simulink model "malt"  (R2022a)
settings: Solver=FixedStepAuto  StartTime=0.0  StopTime=50  FixedStep=framePeriod_s  RelTol=1e-3
undefined symbols (not defined in the file): Aircraft, DiscIntNeverNeededParam, framePeriod_s, frameRate_hz
libraries: simulink x46, slpidlib x16, dspmathops x1
(part 3 of 4)

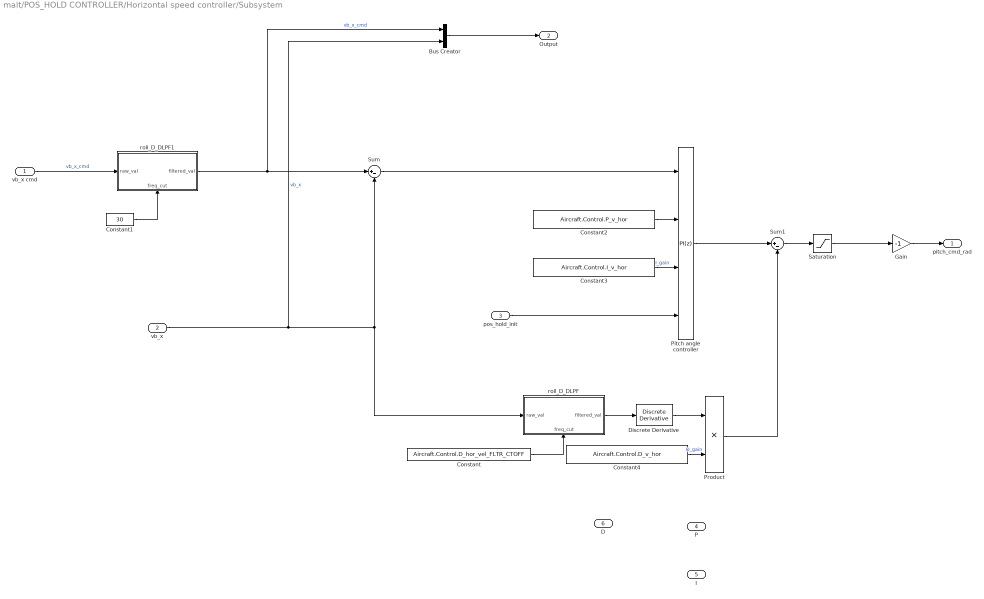
== system malt/POS_HOLD CONTROLLER/Horizontal speed controller/Subsystem ==
  vb_x cmd : Inport
  vb_x : Inport  Port=2
  pos_hold_init : Inport  Port=3
  P : Inport  Port=4
  I : Inport  Port=5
  D : Inport  Port=6
  Bus Creator : BusCreator  Inputs=2
  Constant : Constant  Value=Aircraft.Control.D_hor_vel_FLTR_CTOFF  OutDataTypeStr=single
  Constant1 : Constant  Value=30  OutDataTypeStr=single
  Constant2 : Constant  Value=Aircraft.Control.P_v_hor  OutDataTypeStr=single
  Constant3 : Constant  Value=Aircraft.Control.I_v_hor  OutDataTypeStr=single
  Constant4 : Constant  Value=Aircraft.Control.D_v_hor  OutDataTypeStr=single
  Discrete Derivative : simulink/Discrete/Discrete Derivative  gainval=1.0  ICPrevScaledInput=0.0  OutMin=[]  OutMax=[]  OutDataType=fixdt(1, 16)  OutScaling=2^-10  DoSatur=off
  Gain : Gain  Gain=-1
  Pitch angle controller : slpidlib/PID Controller  Controller=PI  Form=Parallel  TimeDomain=Discrete-time  UseExternalTs=off  SampleTime=framePeriod_s  IntegratorMethod=Forward Euler  FilterMethod=Forward Euler  ControllerParametersSource=external  P=0.335  I=0.005  UseKiTs=off  D=0  N=100  UseFilter=off  TunerSelectOption=Transfer Function Based (PID Tuner App)  InitialConditionSource=internal  InitialConditionForIntegrator=0  InitialConditionForFilter=0  DifferentiatorICPrevScaledInput=0  ExternalReset=either  TrackingMode=off  Kt=1  LimitOutput=on  SatLimitsSource=internal  UpperSaturationLimit=Aircraft.Control.pitch_angle_lim  LowerSaturationLimit=-Aircraft.Control.pitch_angle_lim  LinearizeAsGain=off  AntiWindupMode=clamping  Kb=1  POutMin=[]  POutMax=[]  IOutMin=[]  IOutMax=[]  DOutMin=[]  DOutMax=[]  NOutMin=[]  NOutMax=[]  SumOutMin=[]  SumOutMax=[]  SaturationOutMin=[]  SaturationOutMax=[]  PParamMin=[]  PParamMax=[]  IParamMin=[]  IParamMax=[]  DParamMin=[]  DParamMax=[]  NParamMin=[]  NParamMax=[]  KbParamMin=[]  KbParamMax=[]  KtParamMin=[]  KtParamMax=[]  KbOutMin=[]  KbOutMax=[]  KtOutMin=[]  KtOutMax=[]  IntegratorOutMin=[]  IntegratorOutMax=[]  FilterOutMin=[]  FilterOutMax=[]  SumI1OutMin=[]  SumI1OutMax=[]  SumI2OutMin=[]  SumI2OutMax=[]  SumI3OutMin=[]  SumI3OutMax=[]  SumI4OutMin=[]  SumI4OutMax=[]  SumDOutMin=[]  SumDOutMax=[]  DifferentiatorOutMin=[]  DifferentiatorOutMax=[]  FilterDiffOutCoefMin=[]  FilterDiffOutCoefMax=[]  ReciprocalOutMin=[]  ReciprocalOutMax=[]  SumDenOutMin=[]  SumDenOutMax=[]  SumNumOutMin=[]  SumNumOutMax=[]  DivideOutMin=[]  DivideOutMax=[]  UdiffTsProdOutMin=[]  UdiffTsProdOutMax=[]  NTsProdOutMin=[]  NTsProdOutMax=[]  UintegralTsProdOutMin=[]  UintegralTsProdOutMax=[]  UngainTsProdOutMin=[]  UngainTsProdOutMax=[]  IntegratorContinuousStateAttributes=''  IntegratorStateMustResolveToSignalObject=off  IntegratorRTWStateStorageClass=Auto  FilterContinuousStateAttributes=''  FilterStateMustResolveToSignalObject=off  FilterRTWStateStorageClass=Auto  ParallelPVariant=ExternalParameters  IdealPVariant=Disabled  IVariant=ExternalParameters  DVariant=Disabled  IntegratorVariant=Discrete  SatVariant=Enabled  AWVariant=DiscClampingParallel  PCopyVariant=Disabled  TRVariant=Disabled  FdbkBlocksVariant=Forward  IdealPFdbkVariant=Disabled  SatFdbkVariant=Disabled  DerivativeFilterVariant=Disabled  NVariant=Disabled  NCopyVariant=Disabled_SignalSpec  FilterICVariant=Disabled  IntegratorICVariant=InternalICs  ExternalResetVariant=ExternalReset  TRSumVariant=Passthrough  SumFdbkVariant=Disabled  SumVariant=Sum_PI  TsampFilterVariant=InternalTs  TsampNgainVariant=Passthrough  TsampIntegralVariant=Passthrough  ExternalSaturationOutDataTypeStr=Inherit: Same as second input  aMode=0
  Product : Product
  Saturation : Saturate  UpperLimit=Aircraft.Control.pitch_angle_lim  LowerLimit=-Aircraft.Control.pitch_angle_lim  LinearizeAsGain=off
  Sum : Sum  Inputs=|+-
  Sum1 : Sum  Inputs=|+-
  roll_D_DLPF : Subsystem
      settings: PortSchema="{\"entries\":[{\"content\":{\"sides\":[{\"content\":{\"connectorIds\":[\"In1\"]},\"type\":\"ConnectorPlacement.EquallySpacedRectSide\",\"uuid\":\"20236834-aeb3-4c5b-bb2e-f84447e752b5\"},{\"content\":{\"connectorIds\":[\"Out1\"],\"side\":\"RIGHT\"},\"type\":\"ConnectorPlacement.EquallySpacedRectSide\",\"uuid\":\"d668f9a1-a3df-4207-8bf1-99fb838e59b2\"},{\"content\":{\"connectorIds\":[],\"side\":\"TOP\"},\"type\":\"ConnectorPlacement.EquallySpacedRectSide\",\"uuid\":\"66cceb06-f4bc-4278-b965-2427292e46df\"},{\"content\":{\"connectorIds\":[\"In2\"],\"side\":\"BOTTOM\"},\"type\":\"ConnectorPlacement.EquallySpacedRectSide\",\"uuid\":\"8fdaac6a-cb03-4bd4-87bb-7bafd10bc297\"}]},\"type\":\"ConnectorPlacement.EquallySpacedConnector\",\"uuid\":\"3dc29a9a-e794-478d-b7df-452e6c2d3f66\"}],\"packageUris\":[\"http://schema.mathworks.com/mf0/Connector/R2020b\"],\"version\":\"1.0\"}"
  roll_D_DLPF1 : Subsystem
      settings: PortSchema="{\"entries\":[{\"content\":{\"sides\":[{\"content\":{\"connectorIds\":[\"In1\"]},\"type\":\"ConnectorPlacement.EquallySpacedRectSide\",\"uuid\":\"20236834-aeb3-4c5b-bb2e-f84447e752b5\"},{\"content\":{\"connectorIds\":[\"Out1\"],\"side\":\"RIGHT\"},\"type\":\"ConnectorPlacement.EquallySpacedRectSide\",\"uuid\":\"d668f9a1-a3df-4207-8bf1-99fb838e59b2\"},{\"content\":{\"connectorIds\":[],\"side\":\"TOP\"},\"type\":\"ConnectorPlacement.EquallySpacedRectSide\",\"uuid\":\"66cceb06-f4bc-4278-b965-2427292e46df\"},{\"content\":{\"connectorIds\":[\"In2\"],\"side\":\"BOTTOM\"},\"type\":\"ConnectorPlacement.EquallySpacedRectSide\",\"uuid\":\"8fdaac6a-cb03-4bd4-87bb-7bafd10bc297\"}]},\"type\":\"ConnectorPlacement.EquallySpacedConnector\",\"uuid\":\"3dc29a9a-e794-478d-b7df-452e6c2d3f66\"}],\"packageUris\":[\"http://schema.mathworks.com/mf0/Connector/R2020b\"],\"version\":\"1.0\"}"
  pitch_cmd_rad : Outport
  Output : Outport  Port=2
  wires:
  vb_x/1 -> Bus Creator/2, roll_D_DLPF/1(raw_val), Sum/2  "vb_x"
  Sum/1 -> Pitch angle controller/1
  Saturation/1 -> Gain/1
  Gain/1 -> pitch_cmd_rad/1
  pos_hold_init/1 -> Pitch angle controller/4
  Discrete Derivative/1 -> Product/1
  Constant/1 -> roll_D_DLPF/2(freq_cut)
  roll_D_DLPF/1(filtered_val) -> Discrete Derivative/1
  Pitch angle controller/1 -> Sum1/1
  Sum1/1 -> Saturation/1
  Product/1 -> Sum1/2
  Bus Creator/1 -> Output/1
  vb_x cmd/1 -> roll_D_DLPF1/1(raw_val)  "vb_x_cmd"
  roll_D_DLPF1/1(filtered_val) -> Sum/1, Bus Creator/1  "vb_x_cmd"
  Constant1/1 -> roll_D_DLPF1/2(freq_cut)
  Constant4/1 -> Product/2  "D_gain"
  Constant2/1 -> Pitch angle controller/2
  Constant3/1 -> Pitch angle controller/3  "I_gain"

== system malt/POS_HOLD CONTROLLER/Horizontal speed controller/Subsystem1 ==
  vb_y cmd : Inport
  vb_y : Inport  Port=2
  pos_hold_init : Inport  Port=3
  P : Inport  Port=4
  I : Inport  Port=5
  D : Inport  Port=6
  Bus Creator : BusCreator  Inputs=2
  Constant : Constant  Value=Aircraft.Control.D_hor_vel_FLTR_CTOFF  OutDataTypeStr=single
  Constant1 : Constant  Value=30  OutDataTypeStr=single
  Constant2 : Constant  Value=Aircraft.Control.P_v_hor  OutDataTypeStr=single
  Constant3 : Constant  Value=Aircraft.Control.I_v_hor  OutDataTypeStr=single
  Constant5 : Constant  Value=Aircraft.Control.D_v_hor  OutDataTypeStr=single
  Discrete Derivative : simulink/Discrete/Discrete Derivative  gainval=1.0  ICPrevScaledInput=0.0  OutMin=[]  OutMax=[]  OutDataType=fixdt(1, 16)  OutScaling=2^-10  DoSatur=off
  Product : Product
  Roll angle controller : slpidlib/PID Controller  Controller=PI  Form=Parallel  TimeDomain=Discrete-time  UseExternalTs=off  SampleTime=framePeriod_s  IntegratorMethod=Forward Euler  FilterMethod=Forward Euler  ControllerParametersSource=external  P=0.335  I=0.005  UseKiTs=off  D=0  N=100  UseFilter=off  TunerSelectOption=Transfer Function Based (PID Tuner App)  InitialConditionSource=internal  InitialConditionForIntegrator=0  InitialConditionForFilter=0  DifferentiatorICPrevScaledInput=0  ExternalReset=either  TrackingMode=off  Kt=1  LimitOutput=on  SatLimitsSource=internal  UpperSaturationLimit=Aircraft.Control.roll_angle_lim  LowerSaturationLimit=-Aircraft.Control.roll_angle_lim  LinearizeAsGain=off  AntiWindupMode=clamping  Kb=1  POutMin=[]  POutMax=[]  IOutMin=[]  IOutMax=[]  DOutMin=[]  DOutMax=[]  NOutMin=[]  NOutMax=[]  SumOutMin=[]  SumOutMax=[]  SaturationOutMin=[]  SaturationOutMax=[]  PParamMin=[]  PParamMax=[]  IParamMin=[]  IParamMax=[]  DParamMin=[]  DParamMax=[]  NParamMin=[]  NParamMax=[]  KbParamMin=[]  KbParamMax=[]  KtParamMin=[]  KtParamMax=[]  KbOutMin=[]  KbOutMax=[]  KtOutMin=[]  KtOutMax=[]  IntegratorOutMin=[]  IntegratorOutMax=[]  FilterOutMin=[]  FilterOutMax=[]  SumI1OutMin=[]  SumI1OutMax=[]  SumI2OutMin=[]  SumI2OutMax=[]  SumI3OutMin=[]  SumI3OutMax=[]  SumI4OutMin=[]  SumI4OutMax=[]  SumDOutMin=[]  SumDOutMax=[]  DifferentiatorOutMin=[]  DifferentiatorOutMax=[]  FilterDiffOutCoefMin=[]  FilterDiffOutCoefMax=[]  ReciprocalOutMin=[]  ReciprocalOutMax=[]  SumDenOutMin=[]  SumDenOutMax=[]  SumNumOutMin=[]  SumNumOutMax=[]  DivideOutMin=[]  DivideOutMax=[]  UdiffTsProdOutMin=[]  UdiffTsProdOutMax=[]  NTsProdOutMin=[]  NTsProdOutMax=[]  UintegralTsProdOutMin=[]  UintegralTsProdOutMax=[]  UngainTsProdOutMin=[]  UngainTsProdOutMax=[]  IntegratorContinuousStateAttributes=''  IntegratorStateMustResolveToSignalObject=off  IntegratorRTWStateStorageClass=Auto  FilterContinuousStateAttributes=''  FilterStateMustResolveToSignalObject=off  FilterRTWStateStorageClass=Auto  ParallelPVariant=ExternalParameters  IdealPVariant=Disabled  IVariant=ExternalParameters  DVariant=Disabled  IntegratorVariant=Discrete  SatVariant=Enabled  AWVariant=DiscClampingParallel  PCopyVariant=Disabled  TRVariant=Disabled  FdbkBlocksVariant=Forward  IdealPFdbkVariant=Disabled  SatFdbkVariant=Disabled  DerivativeFilterVariant=Disabled  NVariant=Disabled  NCopyVariant=Disabled_SignalSpec  FilterICVariant=Disabled  IntegratorICVariant=InternalICs  ExternalResetVariant=ExternalReset  TRSumVariant=Passthrough  SumFdbkVariant=Disabled  SumVariant=Sum_PI  TsampFilterVariant=InternalTs  TsampNgainVariant=Passthrough  TsampIntegralVariant=Passthrough  ExternalSaturationOutDataTypeStr=Inherit: Same as second input  aMode=0
  Saturation : Saturate  UpperLimit=Aircraft.Control.pitch_angle_lim  LowerLimit=-Aircraft.Control.pitch_angle_lim  LinearizeAsGain=off
  Sum : Sum  Inputs=|+-
  Sum1 : Sum  Inputs=|+-
  roll_D_DLPF : Subsystem
      settings: PortSchema="{\"entries\":[{\"content\":{\"sides\":[{\"content\":{\"connectorIds\":[\"In1\"]},\"type\":\"ConnectorPlacement.EquallySpacedRectSide\",\"uuid\":\"20236834-aeb3-4c5b-bb2e-f84447e752b5\"},{\"content\":{\"connectorIds\":[\"Out1\"],\"side\":\"RIGHT\"},\"type\":\"ConnectorPlacement.EquallySpacedRectSide\",\"uuid\":\"d668f9a1-a3df-4207-8bf1-99fb838e59b2\"},{\"content\":{\"connectorIds\":[],\"side\":\"TOP\"},\"type\":\"ConnectorPlacement.EquallySpacedRectSide\",\"uuid\":\"66cceb06-f4bc-4278-b965-2427292e46df\"},{\"content\":{\"connectorIds\":[\"In2\"],\"side\":\"BOTTOM\"},\"type\":\"ConnectorPlacement.EquallySpacedRectSide\",\"uuid\":\"8fdaac6a-cb03-4bd4-87bb-7bafd10bc297\"}]},\"type\":\"ConnectorPlacement.EquallySpacedConnector\",\"uuid\":\"3dc29a9a-e794-478d-b7df-452e6c2d3f66\"}],\"packageUris\":[\"http://schema.mathworks.com/mf0/Connector/R2020b\"],\"version\":\"1.0\"}"
  roll_D_DLPF1 : Subsystem
      settings: PortSchema="{\"entries\":[{\"content\":{\"sides\":[{\"content\":{\"connectorIds\":[\"In1\"]},\"type\":\"ConnectorPlacement.EquallySpacedRectSide\",\"uuid\":\"20236834-aeb3-4c5b-bb2e-f84447e752b5\"},{\"content\":{\"connectorIds\":[\"Out1\"],\"side\":\"RIGHT\"},\"type\":\"ConnectorPlacement.EquallySpacedRectSide\",\"uuid\":\"d668f9a1-a3df-4207-8bf1-99fb838e59b2\"},{\"content\":{\"connectorIds\":[],\"side\":\"TOP\"},\"type\":\"ConnectorPlacement.EquallySpacedRectSide\",\"uuid\":\"66cceb06-f4bc-4278-b965-2427292e46df\"},{\"content\":{\"connectorIds\":[\"In2\"],\"side\":\"BOTTOM\"},\"type\":\"ConnectorPlacement.EquallySpacedRectSide\",\"uuid\":\"8fdaac6a-cb03-4bd4-87bb-7bafd10bc297\"}]},\"type\":\"ConnectorPlacement.EquallySpacedConnector\",\"uuid\":\"3dc29a9a-e794-478d-b7df-452e6c2d3f66\"}],\"packageUris\":[\"http://schema.mathworks.com/mf0/Connector/R2020b\"],\"version\":\"1.0\"}"
  roll_cmd_rad : Outport
  Output : Outport  Port=2
  wires:
  vb_y/1 -> Bus Creator/2, roll_D_DLPF/1(raw_val), Sum/2  "vb_y"
  Sum/1 -> Roll angle controller/1
  Saturation/1 -> roll_cmd_rad/1
  pos_hold_init/1 -> Roll angle controller/4
  Discrete Derivative/1 -> Product/1
  Constant/1 -> roll_D_DLPF/2(freq_cut)
  roll_D_DLPF/1(filtered_val) -> Discrete Derivative/1
  Roll angle controller/1 -> Sum1/1
  Sum1/1 -> Saturation/1
  Product/1 -> Sum1/2
  Bus Creator/1 -> Output/1
  vb_y cmd/1 -> roll_D_DLPF1/1(raw_val)  "vb_x_cmd"
  Constant1/1 -> roll_D_DLPF1/2(freq_cut)
  roll_D_DLPF1/1(filtered_val) -> Sum/1, Bus Creator/1  "vb_y_cmd"
  Constant5/1 -> Product/2  "I_gain"
  Constant2/1 -> Roll angle controller/2
  Constant3/1 -> Roll angle controller/3  "I_gain"

== system malt/POS_HOLD CONTROLLER/Horizontal speed controller/zero_vel_handling ==
  vb_x cmd : Inport
  vb_y_cmd : Inport  Port=2
  pos_e_feedback : Inport  Port=3
  cur_heading_rad : Inport  Port=4
  pos_hold_init : Inport  Port=5
  P : Inport  Port=6
  AND : Logic  IconShape=distinctive  AllPortsSameDT=off  OutDataTypeStr=boolean
  Cast To Single : DataTypeConversion  OutDataTypeStr=single  SaturateOnIntegerOverflow=off  RndMeth=Floor
  Compare To Constant : simulink/Logic and Bit Operations/Compare To Constant  relop===  const=0  OutDataTypeStr=boolean
  Compare To Constant1 : simulink/Logic and Bit Operations/Compare To Constant  relop===  const=0  OutDataTypeStr=boolean
  Detect Change : simulink/Logic and Bit Operations/Detect Change  vinit=0  OutDataTypeStr=boolean
  Horizontal position controller : Subsystem
  Mux : Mux  Inputs=2
  Mux1 : Mux  Inputs=2
  NOT : Logic  Operator=NOT  IconShape=distinctive  AllPortsSameDT=off  OutDataTypeStr=boolean
  OR : Logic  Operator=OR  IconShape=distinctive  AllPortsSameDT=off  OutDataTypeStr=boolean
  Switch : Switch  Criteria=u2 > Threshold  SaturateOnIntegerOverflow=off  InputSameDT=off
  Unit Delay : UnitDelay  SampleTime=-1  HasFrameUpgradeWarning=on
  set_tar_pos when vel_cmd == 0 : Subsystem  TreatAsAtomicUnit=on
  v_cmd : Outport
  tar_pos_pos_hold : Outport  Port=2
  wires:
  Mux/1 -> Switch/1
  vb_y_cmd/1 -> Mux/2, Compare To Constant1/1
  Compare To Constant1/1 -> AND/2
  Switch/1 -> v_cmd/1
  vb_x cmd/1 -> Mux/1, Compare To Constant/1
  Compare To Constant/1 -> AND/1
  NOT/1 -> set_tar_pos when vel_cmd == 0/Enable, Switch/2
  pos_e_feedback/1 -> set_tar_pos when vel_cmd == 0/1(pos_xy_m), Horizontal position controller/2(cur_pos_m)
  Horizontal position controller/1(vb_x_cmd_mps) -> Mux1/1  "vb_x_cmd_mps"
  Horizontal position controller/2(vb_y_cmd_mps) -> Mux1/2  "vb_y_cmd_mps"
  cur_heading_rad/1 -> Horizontal position controller/3(cur_heading_rad)
  Mux1/1 -> Cast To Single/1
  Cast To Single/1 -> Switch/3
  OR/1 -> NOT/1
  AND/1 -> OR/1
  pos_hold_init/1 -> Unit Delay/1
  Detect Change/1 -> OR/2
  Unit Delay/1 -> Detect Change/1
  set_tar_pos when vel_cmd == 0/1(target_pos_xy_m) -> tar_pos_pos_hold/1, Horizontal position controller/1(cur_target_pos_m)
  P/1 -> Horizontal position controller/4(P)

== system malt/POS_HOLD CONTROLLER/Vertical speed controller/Pitch_D_DLPF ==
  raw_val : Inport
  freq_cut : Inport  Port=2
  MATLAB Function : MATLAB Function  TreatAsAtomicUnit=on
  Unit Delay : UnitDelay  SampleTime=-1  HasFrameUpgradeWarning=on
  filtered_val : Outport
  wires:
  MATLAB Function/1(filtered_val) -> filtered_val/1, Unit Delay/1
  raw_val/1 -> MATLAB Function/2(raw_val)
  Unit Delay/1 -> MATLAB Function/1(prev_val)
  freq_cut/1 -> MATLAB Function/3(freq_cut)

== system malt/POS_HOLD CONTROLLER/Vertical speed controller/Vertical position controller ==
  cur_alt : Inport
  tar_z : Inport  Port=2
  P_alt : Inport  Port=3
  Altitude PID : slpidlib/PID Controller  Controller=P  Form=Ideal  TimeDomain=Discrete-time  UseExternalTs=off  SampleTime=framePeriod_s  IntegratorMethod=Forward Euler  FilterMethod=Forward Euler  ControllerParametersSource=external  P=0  I=0  UseKiTs=off  D=0  N=100  UseFilter=off  TunerSelectOption=Frequency Response Based  ZeroCross=off  InitialConditionSource=internal  InitialConditionForIntegrator=0  InitialConditionForFilter=0  DifferentiatorICPrevScaledInput=0  ExternalReset=either  TrackingMode=off  Kt=1  LimitOutput=on  SatLimitsSource=internal  UpperSaturationLimit=Aircraft.Control.v_z_up_max  LowerSaturationLimit=-Aircraft.Control.v_z_down_max  LinearizeAsGain=on  AntiWindupMode=clamping  Kb=1  POutMin=[]  POutMax=[]  IOutMin=[]  IOutMax=[]  DOutMin=[]  DOutMax=[]  NOutMin=[]  NOutMax=[]  SumOutMin=[]  SumOutMax=[]  SaturationOutMin=[]  SaturationOutMax=[]  PParamMin=[]  PParamMax=[]  IParamMin=[]  IParamMax=[]  DParamMin=[]  DParamMax=[]  NParamMin=[]  NParamMax=[]  KbParamMin=[]  KbParamMax=[]  KtParamMin=[]  KtParamMax=[]  KbOutMin=[]  KbOutMax=[]  KtOutMin=[]  KtOutMax=[]  IntegratorOutMin=[]  IntegratorOutMax=[]  FilterOutMin=[]  FilterOutMax=[]  SumI1OutMin=[]  SumI1OutMax=[]  SumI2OutMin=[]  SumI2OutMax=[]  SumI3OutMin=[]  SumI3OutMax=[]  SumI4OutMin=[]  SumI4OutMax=[]  SumDOutMin=[]  SumDOutMax=[]  DifferentiatorOutMin=[]  DifferentiatorOutMax=[]  FilterDiffOutCoefMin=[]  FilterDiffOutCoefMax=[]  ReciprocalOutMin=[]  ReciprocalOutMax=[]  SumDenOutMin=[]  SumDenOutMax=[]  SumNumOutMin=[]  SumNumOutMax=[]  DivideOutMin=[]  DivideOutMax=[]  UdiffTsProdOutMin=[]  UdiffTsProdOutMax=[]  NTsProdOutMin=[]  NTsProdOutMax=[]  UintegralTsProdOutMin=[]  UintegralTsProdOutMax=[]  UngainTsProdOutMin=[]  UngainTsProdOutMax=[]  IntegratorContinuousStateAttributes=''  IntegratorStateMustResolveToSignalObject=off  IntegratorRTWStateStorageClass=Auto  FilterContinuousStateAttributes=''  FilterStateMustResolveToSignalObject=off  FilterRTWStateStorageClass=Auto  ParallelPVariant=ExternalParameters  IdealPVariant=Disabled  IVariant=Disabled  DVariant=Disabled  IntegratorVariant=Disabled  SatVariant=Enabled  AWVariant=Disabled  PCopyVariant=Disabled  TRVariant=Disabled  FdbkBlocksVariant=Forward  IdealPFdbkVariant=Disabled  SatFdbkVariant=Disabled  DerivativeFilterVariant=Disabled  NVariant=Disabled  NCopyVariant=Disabled_SignalSpec  FilterICVariant=Disabled  IntegratorICVariant=Disabled  ExternalResetVariant=Disabled  TRSumVariant=Passthrough  SumFdbkVariant=Disabled  SumVariant=Passthrough_P  TsampFilterVariant=InternalTs  TsampNgainVariant=Passthrough  TsampIntegralVariant=Disabled_SignalSpec  ExternalSaturationOutDataTypeStr=Inherit: Same as second input  aMode=0
  Sum3 : Sum  Inputs=|+-
  ve_z_cmd_mps : Outport
  wires:
  Altitude PID/1 -> ve_z_cmd_mps/1
  tar_z/1 -> Sum3/1  "target_z"
  cur_alt/1 -> Sum3/2
  Sum3/1 -> Altitude PID/1
  P_alt/1 -> Altitude PID/2

== system malt/POS_HOLD CONTROLLER/Vertical speed controller/set_tar_z when ve_z_cmd == 0 ==
  In1 : Inport
  Enable : EnablePort
  tar_z : Outport
  wires:
  In1/1 -> tar_z/1

== system malt/WAYPOINT CONTROLLER1/WP_NAV/Horizontal position controller ==
  Sys_input : Inport
  cur_target_pos_m : Inport  Port=2
  prev_pos_m : Inport  Port=3
  Bus Creator : BusCreator  Inputs=2
  Bus Selector2 : BusSelector  OutputSignals=Aux Ins Data.ned_pos_m,Ins Data.heading_rad
  Horizontal_position_controller : Subsystem
  deviation_calc : MATLAB Function  TreatAsAtomicUnit=on
  "horizontal_error_calculation " : Subsystem
  vb_x_cmd_mps : Outport
  vb_y_cmd_mps : Outport  Port=2
  Output : Outport  Port=3
  Output1 : Outport  Port=4
  wires:
  Horizontal_position_controller/1(vb_x) -> vb_x_cmd_mps/1
  Horizontal_position_controller/2(vb_y) -> vb_y_cmd_mps/1
  Sys_input/1 -> Bus Selector2/1
  "horizontal_error_calculation "/1(dist_to_target_m) -> Horizontal_position_controller/1(dist_to_tar_m)
  "horizontal_error_calculation "/2(bearing_to_tar_rad) -> Horizontal_position_controller/2(bearing_to_tar_rad)
  Bus Selector2/1 -> "horizontal_error_calculation "/2(cur_pos_m), deviation_calc/2(cur_pos)  "<ned_pos_m>"
  Bus Selector2/2 -> Horizontal_position_controller/5(cur_heading_rad)  "<heading_rad>"
  deviation_calc/1(dev_dist_m) -> Horizontal_position_controller/3(dev_dist_m), Bus Creator/1  "dev_dist"
  cur_target_pos_m/1 -> deviation_calc/1(tar_pos), "horizontal_error_calculation "/1(target_pos_m)
  prev_pos_m/1 -> deviation_calc/3(prev_pos)
  deviation_calc/2(dev_bearing_rad) -> Horizontal_position_controller/4(dev_bearing_rad), Bus Creator/2  "dev_bearing"
  Bus Creator/1 -> Output/1
  Horizontal_position_controller/3(dev_output) -> Output1/1

== system malt/WAYPOINT CONTROLLER1/WP_NAV/Vertical position controller ==
  Sys_input : Inport
  max_v_z_mps : Inport  Port=2
  cur_target_pos_m : Inport  Port=3
  Bus Selector6 : BusSelector  OutputSignals=Navigation Filter Data.bfs_ekf.ned_pos_m
  Selector1 : Selector  InputPortWidth=3  IndexOptions=Index vector (dialog)  Indices=3  OutputSizes=1
  select_cur_z : Selector  InputPortWidth=3  IndexOptions=Index vector (dialog)  Indices=3  OutputSizes=1
  vertical_position_controller : Subsystem
  ve_z_cmd_mps : Outport
  wires:
  Sys_input/1 -> Bus Selector6/1
  Bus Selector6/1 -> select_cur_z/1  "<ned_pos_m>"
  vertical_position_controller/1(ve_z_cmd) -> ve_z_cmd_mps/1
  Selector1/1 -> vertical_position_controller/1(target_z_m)  "target_z"
  select_cur_z/1 -> vertical_position_controller/2(cur_z_m)
  cur_target_pos_m/1 -> Selector1/1
  max_v_z_mps/1 -> vertical_position_controller/3(max_v_z_mps)

== system malt/WAYPOINT CONTROLLER1/WP_NAV/heading_controller ==
  Sys_input : Inport
  cur_target_heading_rad : Inport  Port=2
  Bus Selector4 : BusSelector  OutputSignals=Navigation Filter Data.bfs_ekf.heading_rad
  heading_controller : Subsystem
  yaw_rate_cmd_radps : Outport
  wires:
  Sys_input/1 -> Bus Selector4/1
  cur_target_heading_rad/1 -> heading_controller/1(heading_cmd_rad)
  Bus Selector4/1 -> heading_controller/2(<heading_rad>)  "<heading_rad>"
  heading_controller/1(yaw_rate_cmd) -> yaw_rate_cmd_radps/1

== system malt/determine arm and mode selection/Failsafe_management/Radio failsafe ==
  note: Transition to RTL mode
  note: If radio_failsafe is triggered and current_mode is not auto, rtl, land nor motor_state disarmed then RTL mode is triggered
  failsafe : Inport
  manual_mode : Inport  Port=2
  motor_state : Inport  Port=3
  AND1 : Logic  Commented=on  IconShape=distinctive  AllPortsSameDT=off  OutDataTypeStr=boolean
  Compare To Constant : simulink/Logic and Bit Operations/Compare To Constant  Commented=on  relop=~=  const=3  OutDataTypeStr=boolean
  Compare To Constant1 : simulink/Logic and Bit Operations/Compare To Constant  Commented=on  relop=~=  const=4  OutDataTypeStr=boolean
  Compare To Constant2 : simulink/Logic and Bit Operations/Compare To Constant  Commented=on  relop=~=  const=5  OutDataTypeStr=boolean
  NOR : Logic  Commented=on  Operator=NOR  Inputs=4  IconShape=distinctive  AllPortsSameDT=off  OutDataTypeStr=boolean
  NOT : Logic  Commented=on  Operator=NOT  IconShape=distinctive  AllPortsSameDT=off  OutDataTypeStr=boolean
  NOT1 : Logic  Operator=NOT  IconShape=distinctive  AllPortsSameDT=off  OutDataTypeStr=boolean
  Subsystem : Subsystem
  radio_failsafe_enabled : Outport
  wires:
  manual_mode/1 -> Compare To Constant2/1, Compare To Constant1/1, Compare To Constant/1
  Compare To Constant/1 -> NOR/1
  Compare To Constant1/1 -> NOR/2
  Compare To Constant2/1 -> NOR/3
  motor_state/1 -> NOT/1
  NOT/1 -> NOR/4
  failsafe/1 -> Subsystem/1(<inceptor_health>)
  NOR/1 -> AND1/1
  Subsystem/1(inceptor_health_filtered) -> NOT1/1
  NOT1/1 -> radio_failsafe_enabled/1

== system malt/determine arm and mode selection/Subsystem/e_stop counter ==
  note: This is to ensure e_stop event is not triggered unless e_stop command is sent for more than 0.3 s to prevent false trigger
  motor_e_stop_raw : Inport
  Enable : EnablePort  StatesWhenEnabling=reset
  Compare To Constant : simulink/Logic and Bit Operations/Compare To Constant  relop=>=  const=0.5  OutDataTypeStr=boolean
  Discrete-Time Integrator : DiscreteIntegrator  SampleTime=framePeriod_s  LimitOutput=on  UpperSaturationLimit=1  LowerSaturationLimit=0  ICPrevOutput=DiscIntNeverNeededParam  ICPrevScaledInput=DiscIntNeverNeededParam
  Gain : Gain  Gain=2
  e_stop_filtered : Outport
  wires:
  Compare To Constant/1 -> e_stop_filtered/1
  Discrete-Time Integrator/1 -> Compare To Constant/1
  Gain/1 -> Discrete-Time Integrator/1
  motor_e_stop_raw/1 -> Gain/1

== system malt/determine arm and mode selection/yaw_stick_arming/Enabled Subsystem ==
  yaw_input : Inport
  Enable : EnablePort  StatesWhenEnabling=reset
  Cast : DataTypeConversion  OutDataTypeStr=int8  SaturateOnIntegerOverflow=off  RndMeth=Floor
  Discrete-Time Integrator : DiscreteIntegrator  IntegratorMethod=Integration: Trapezoidal  SampleTime=framePeriod_s  OutDataTypeStr=single  UpperSaturationLimit=1  LowerSaturationLimit=0  ICPrevOutput=DiscIntNeverNeededParam  ICPrevScaledInput=DiscIntNeverNeededParam
  time_arm_valid_s : Outport
  wires:
  Discrete-Time Integrator/1 -> time_arm_valid_s/1
  Cast/1 -> Discrete-Time Integrator/1
  yaw_input/1 -> Cast/1

== system malt/determine arm and mode selection/yaw_stick_arming/manual_arming ==
  yaw_arm : Inport
  Trigger : TriggerPort  VariantControl=(inherit)  PortDimensions=1
  arm_state : Outport
  wires:
  yaw_arm/1 -> arm_state/1

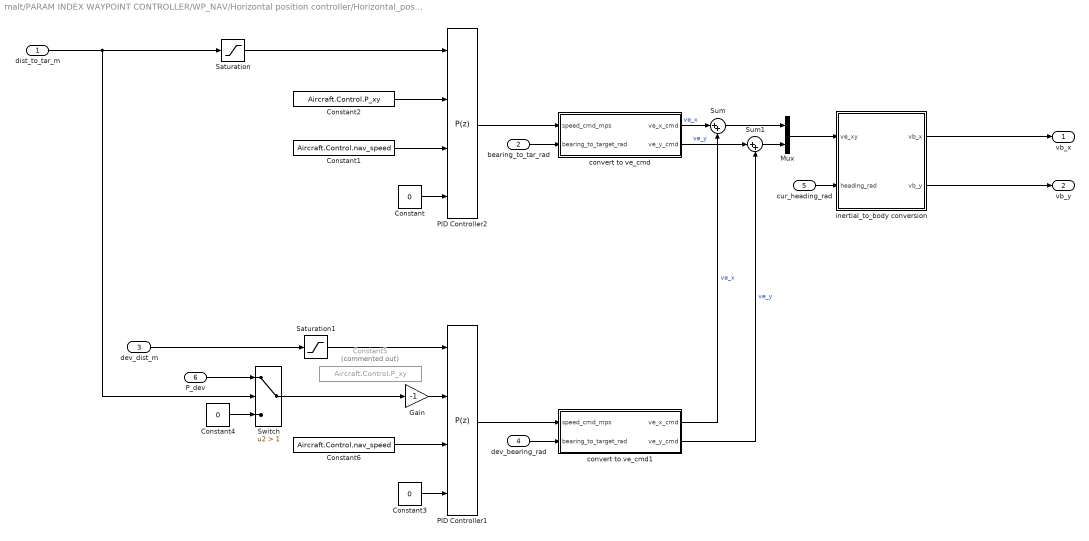
== system malt/PARAM INDEX WAYPOINT CONTROLLER/WP_NAV/Horizontal position controller/Horizontal_position_controller ==
  dist_to_tar_m : Inport
  bearing_to_tar_rad : Inport  Port=2
  dev_dist_m : Inport  Port=3
  dev_bearing_rad : Inport  Port=4
  cur_heading_rad : Inport  Port=5
  P_dev : Inport  Port=6
  Constant : Constant  Value=0  OutDataTypeStr=single
  Constant1 : Constant  Value=Aircraft.Control.nav_speed  OutDataTypeStr=single
  Constant2 : Constant  Value=Aircraft.Control.P_xy  OutDataTypeStr=single
  Constant3 : Constant  Value=0  OutDataTypeStr=single
  Constant4 : Constant  Value=0  OutDataTypeStr=single
  Constant5 : Constant  Commented=on  Value=Aircraft.Control.P_xy  OutDataTypeStr=single
  Constant6 : Constant  Value=Aircraft.Control.nav_speed  OutDataTypeStr=single
  Gain : Gain  Gain=-1
  Mux : Mux  Inputs=2
  PID Controller1 : slpidlib/PID Controller  Controller=P  Form=Parallel  TimeDomain=Discrete-time  UseExternalTs=off  SampleTime=framePeriod_s  IntegratorMethod=Forward Euler  FilterMethod=Forward Euler  ControllerParametersSource=external  P=0.335  I=0.005  UseKiTs=off  D=0  N=100  UseFilter=off  TunerSelectOption=Transfer Function Based (PID Tuner App)  InitialConditionSource=internal  InitialConditionForIntegrator=0  InitialConditionForFilter=0  DifferentiatorICPrevScaledInput=0  ExternalReset=none  TrackingMode=off  Kt=1  LimitOutput=on  SatLimitsSource=external  UpperSaturationLimit=inf  LowerSaturationLimit=-inf  LinearizeAsGain=off  AntiWindupMode=clamping  Kb=1  POutMin=[]  POutMax=[]  IOutMin=[]  IOutMax=[]  DOutMin=[]  DOutMax=[]  NOutMin=[]  NOutMax=[]  SumOutMin=[]  SumOutMax=[]  SaturationOutMin=[]  SaturationOutMax=[]  PParamMin=[]  PParamMax=[]  IParamMin=[]  IParamMax=[]  DParamMin=[]  DParamMax=[]  NParamMin=[]  NParamMax=[]  KbParamMin=[]  KbParamMax=[]  KtParamMin=[]  KtParamMax=[]  KbOutMin=[]  KbOutMax=[]  KtOutMin=[]  KtOutMax=[]  IntegratorOutMin=[]  IntegratorOutMax=[]  FilterOutMin=[]  FilterOutMax=[]  SumI1OutMin=[]  SumI1OutMax=[]  SumI2OutMin=[]  SumI2OutMax=[]  SumI3OutMin=[]  SumI3OutMax=[]  SumI4OutMin=[]  SumI4OutMax=[]  SumDOutMin=[]  SumDOutMax=[]  DifferentiatorOutMin=[]  DifferentiatorOutMax=[]  FilterDiffOutCoefMin=[]  FilterDiffOutCoefMax=[]  ReciprocalOutMin=[]  ReciprocalOutMax=[]  SumDenOutMin=[]  SumDenOutMax=[]  SumNumOutMin=[]  SumNumOutMax=[]  DivideOutMin=[]  DivideOutMax=[]  UdiffTsProdOutMin=[]  UdiffTsProdOutMax=[]  NTsProdOutMin=[]  NTsProdOutMax=[]  UintegralTsProdOutMin=[]  UintegralTsProdOutMax=[]  UngainTsProdOutMin=[]  UngainTsProdOutMax=[]  IntegratorContinuousStateAttributes=''  IntegratorStateMustResolveToSignalObject=off  IntegratorRTWStateStorageClass=Auto  FilterContinuousStateAttributes=''  FilterStateMustResolveToSignalObject=off  FilterRTWStateStorageClass=Auto  ParallelPVariant=ExternalParameters  IdealPVariant=Disabled  IVariant=Disabled  DVariant=Disabled  IntegratorVariant=Disabled  SatVariant=External  AWVariant=Disabled  PCopyVariant=Disabled  TRVariant=Disabled  FdbkBlocksVariant=Forward  IdealPFdbkVariant=Disabled  SatFdbkVariant=Disabled  DerivativeFilterVariant=Disabled  NVariant=Disabled  NCopyVariant=Disabled_SignalSpec  FilterICVariant=Disabled  IntegratorICVariant=Disabled  ExternalResetVariant=Disabled  TRSumVariant=Passthrough  SumFdbkVariant=Disabled  SumVariant=Passthrough_P  TsampFilterVariant=InternalTs  TsampNgainVariant=Passthrough  TsampIntegralVariant=Disabled_SignalSpec  ExternalSaturationOutDataTypeStr=Inherit: Same as second input  aMode=0
  PID Controller2 : slpidlib/PID Controller  Controller=P  Form=Parallel  TimeDomain=Discrete-time  UseExternalTs=off  SampleTime=framePeriod_s  IntegratorMethod=Forward Euler  FilterMethod=Forward Euler  ControllerParametersSource=external  P=0.335  I=0.005  UseKiTs=off  D=0  N=100  UseFilter=off  TunerSelectOption=Transfer Function Based (PID Tuner App)  InitialConditionSource=internal  InitialConditionForIntegrator=0  InitialConditionForFilter=0  DifferentiatorICPrevScaledInput=0  ExternalReset=none  TrackingMode=off  Kt=1  LimitOutput=on  SatLimitsSource=external  UpperSaturationLimit=inf  LowerSaturationLimit=-inf  LinearizeAsGain=off  AntiWindupMode=clamping  Kb=1  POutMin=[]  POutMax=[]  IOutMin=[]  IOutMax=[]  DOutMin=[]  DOutMax=[]  NOutMin=[]  NOutMax=[]  SumOutMin=[]  SumOutMax=[]  SaturationOutMin=[]  SaturationOutMax=[]  PParamMin=[]  PParamMax=[]  IParamMin=[]  IParamMax=[]  DParamMin=[]  DParamMax=[]  NParamMin=[]  NParamMax=[]  KbParamMin=[]  KbParamMax=[]  KtParamMin=[]  KtParamMax=[]  KbOutMin=[]  KbOutMax=[]  KtOutMin=[]  KtOutMax=[]  IntegratorOutMin=[]  IntegratorOutMax=[]  FilterOutMin=[]  FilterOutMax=[]  SumI1OutMin=[]  SumI1OutMax=[]  SumI2OutMin=[]  SumI2OutMax=[]  SumI3OutMin=[]  SumI3OutMax=[]  SumI4OutMin=[]  SumI4OutMax=[]  SumDOutMin=[]  SumDOutMax=[]  DifferentiatorOutMin=[]  DifferentiatorOutMax=[]  FilterDiffOutCoefMin=[]  FilterDiffOutCoefMax=[]  ReciprocalOutMin=[]  ReciprocalOutMax=[]  SumDenOutMin=[]  SumDenOutMax=[]  SumNumOutMin=[]  SumNumOutMax=[]  DivideOutMin=[]  DivideOutMax=[]  UdiffTsProdOutMin=[]  UdiffTsProdOutMax=[]  NTsProdOutMin=[]  NTsProdOutMax=[]  UintegralTsProdOutMin=[]  UintegralTsProdOutMax=[]  UngainTsProdOutMin=[]  UngainTsProdOutMax=[]  IntegratorContinuousStateAttributes=''  IntegratorStateMustResolveToSignalObject=off  IntegratorRTWStateStorageClass=Auto  FilterContinuousStateAttributes=''  FilterStateMustResolveToSignalObject=off  FilterRTWStateStorageClass=Auto  ParallelPVariant=ExternalParameters  IdealPVariant=Disabled  IVariant=Disabled  DVariant=Disabled  IntegratorVariant=Disabled  SatVariant=External  AWVariant=Disabled  PCopyVariant=Disabled  TRVariant=Disabled  FdbkBlocksVariant=Forward  IdealPFdbkVariant=Disabled  SatFdbkVariant=Disabled  DerivativeFilterVariant=Disabled  NVariant=Disabled  NCopyVariant=Disabled_SignalSpec  FilterICVariant=Disabled  IntegratorICVariant=Disabled  ExternalResetVariant=Disabled  TRSumVariant=Passthrough  SumFdbkVariant=Disabled  SumVariant=Passthrough_P  TsampFilterVariant=InternalTs  TsampNgainVariant=Passthrough  TsampIntegralVariant=Disabled_SignalSpec  ExternalSaturationOutDataTypeStr=Inherit: Same as second input  aMode=0
  Saturation : Saturate  UpperLimit=1  LowerLimit=0
  Saturation1 : Saturate  UpperLimit=1  LowerLimit=0
  Sum : Sum  Inputs=|++
  Sum1 : Sum  Inputs=|++
  Switch : Switch  Criteria=u2 > Threshold  Threshold=1  SaturateOnIntegerOverflow=off  InputSameDT=off
  convert to ve_cmd : Subsystem
  convert to ve_cmd1 : Subsystem
  inertial_to_body conversion : Subsystem
  vb_x : Outport
  vb_y : Outport  Port=2
  wires:
  Constant2/1 -> PID Controller2/2
  bearing_to_tar_rad/1 -> convert to ve_cmd/2(bearing_to_target_rad)
  Mux/1 -> inertial_to_body conversion/1(ve_xy)
  Constant1/1 -> PID Controller2/3
  Constant/1 -> PID Controller2/4
  Saturation/1 -> PID Controller2/1
  dist_to_tar_m/1 -> Saturation/1, Switch/2
  cur_heading_rad/1 -> inertial_to_body conversion/2(heading_rad)
  PID Controller2/1 -> convert to ve_cmd/1(speed_cmd_mps)
  inertial_to_body conversion/1(vb_x) -> vb_x/1
  inertial_to_body conversion/2(vb_y) -> vb_y/1
  dev_dist_m/1 -> Saturation1/1
  PID Controller1/1 -> convert to ve_cmd1/1(speed_cmd_mps)
  dev_bearing_rad/1 -> convert to ve_cmd1/2(bearing_to_target_rad)
  Saturation1/1 -> PID Controller1/1
  Constant3/1 -> PID Controller1/4
  Constant6/1 -> PID Controller1/3
  convert to ve_cmd/1(ve_x_cmd) -> Sum/1  "ve_x"
  Sum/1 -> Mux/1
  convert to ve_cmd/2(ve_y_cmd) -> Sum1/1  "ve_y"
  Sum1/1 -> Mux/2
  convert to ve_cmd1/1(ve_x_cmd) -> Sum/2  "ve_x"
  convert to ve_cmd1/2(ve_y_cmd) -> Sum1/2  "ve_y"
  Gain/1 -> PID Controller1/2
  Switch/1 -> Gain/1
  P_dev/1 -> Switch/1
  Constant4/1 -> Switch/3

== system malt/PARAM INDEX WAYPOINT CONTROLLER/WP_NAV/Horizontal position controller/horizontal_error_calculation  ==
  target_pos_m : Inport
  cur_pos_m : Inport  Port=2
  Atan2 : Trigonometry  Operator=atan2
  Demux2 : Demux  Outputs=2
  MatrixMultiply : Product  Multiplication=Matrix(*)
  Selector : Selector  InputPortWidth=3  IndexOptions=Index vector (dialog)  Indices=[1 2]  OutputSizes=1
  Sqrt : Sqrt
  Subtract : Sum  Inputs=+-
  Transpose : Math  Operator=transpose
  dist_to_target_m : Outport
  bearing_to_tar_rad : Outport  Port=2
  wires:
  target_pos_m/1 -> Subtract/1
  cur_pos_m/1 -> Subtract/2
  Selector/1 -> Demux2/1, MatrixMultiply/2, Transpose/1
  Atan2/1 -> bearing_to_tar_rad/1
  Subtract/1 -> Selector/1
  Demux2/2 -> Atan2/1
  Transpose/1 -> MatrixMultiply/1
  MatrixMultiply/1 -> Sqrt/1
  Demux2/1 -> Atan2/2
  Sqrt/1 -> dist_to_target_m/1

== system malt/PARAM INDEX WAYPOINT CONTROLLER/WP_NAV/Vertical position controller/vertical_position_controller ==
  target_z_m : Inport
  cur_z_m : Inport  Port=2
  max_v_z_mps : Inport  Port=3
  Altitude PID : slpidlib/PID Controller  Controller=PI  Form=Ideal  TimeDomain=Discrete-time  UseExternalTs=off  SampleTime=framePeriod_s  IntegratorMethod=Forward Euler  FilterMethod=Forward Euler  ControllerParametersSource=external  P=0  I=0  UseKiTs=off  D=0  N=100  UseFilter=off  TunerSelectOption=Frequency Response Based  ZeroCross=off  InitialConditionSource=internal  InitialConditionForIntegrator=0  InitialConditionForFilter=0  DifferentiatorICPrevScaledInput=0  ExternalReset=none  TrackingMode=off  Kt=1  LimitOutput=on  SatLimitsSource=external  UpperSaturationLimit=Aircraft.Control.v_z_up_max  LowerSaturationLimit=-Aircraft.Control.v_z_down_max  LinearizeAsGain=on  AntiWindupMode=clamping  Kb=1  POutMin=[]  POutMax=[]  IOutMin=[]  IOutMax=[]  DOutMin=[]  DOutMax=[]  NOutMin=[]  NOutMax=[]  SumOutMin=[]  SumOutMax=[]  SaturationOutMin=[]  SaturationOutMax=[]  PParamMin=[]  PParamMax=[]  IParamMin=[]  IParamMax=[]  DParamMin=[]  DParamMax=[]  NParamMin=[]  NParamMax=[]  KbParamMin=[]  KbParamMax=[]  KtParamMin=[]  KtParamMax=[]  KbOutMin=[]  KbOutMax=[]  KtOutMin=[]  KtOutMax=[]  IntegratorOutMin=[]  IntegratorOutMax=[]  FilterOutMin=[]  FilterOutMax=[]  SumI1OutMin=[]  SumI1OutMax=[]  SumI2OutMin=[]  SumI2OutMax=[]  SumI3OutMin=[]  SumI3OutMax=[]  SumI4OutMin=[]  SumI4OutMax=[]  SumDOutMin=[]  SumDOutMax=[]  DifferentiatorOutMin=[]  DifferentiatorOutMax=[]  FilterDiffOutCoefMin=[]  FilterDiffOutCoefMax=[]  ReciprocalOutMin=[]  ReciprocalOutMax=[]  SumDenOutMin=[]  SumDenOutMax=[]  SumNumOutMin=[]  SumNumOutMax=[]  DivideOutMin=[]  DivideOutMax=[]  UdiffTsProdOutMin=[]  UdiffTsProdOutMax=[]  NTsProdOutMin=[]  NTsProdOutMax=[]  UintegralTsProdOutMin=[]  UintegralTsProdOutMax=[]  UngainTsProdOutMin=[]  UngainTsProdOutMax=[]  IntegratorContinuousStateAttributes=''  IntegratorStateMustResolveToSignalObject=off  IntegratorRTWStateStorageClass=Auto  FilterContinuousStateAttributes=''  FilterStateMustResolveToSignalObject=off  FilterRTWStateStorageClass=Auto  ParallelPVariant=Passthrough  IdealPVariant=ExternalParameters  IVariant=ExternalParameters  DVariant=Disabled  IntegratorVariant=Discrete  SatVariant=External  AWVariant=DiscClampingIdeal  PCopyVariant=ExternalParamsIdeal  TRVariant=Disabled  FdbkBlocksVariant=Forward  IdealPFdbkVariant=Disabled  SatFdbkVariant=Disabled  DerivativeFilterVariant=Disabled  NVariant=Disabled  NCopyVariant=Disabled_SignalSpec  FilterICVariant=Disabled  IntegratorICVariant=InternalICs  ExternalResetVariant=Disabled  TRSumVariant=Passthrough  SumFdbkVariant=Disabled  SumVariant=Sum_PI  TsampFilterVariant=InternalTs  TsampNgainVariant=Passthrough  TsampIntegralVariant=Passthrough  ExternalSaturationOutDataTypeStr=Inherit: Same as second input  aMode=0
  Constant : Constant  Value=Aircraft.Control.v_z_up_max  OutDataTypeStr=single
  Constant1 : Constant  Value=Aircraft.Control.v_z_down_max  OutDataTypeStr=single
  Gain : Gain  Gain=-1
  Min : MinMax  Inputs=2
  P_alt : Constant  Value=Aircraft.Control.P_alt  OutDataTypeStr=single
  P_alt1 : Constant  Value=Aircraft.Control.I_alt  OutDataTypeStr=single
  Sum3 : Sum  Inputs=|+-
  ve_z_cmd : Outport
  wires:
  P_alt/1 -> Altitude PID/2
  Sum3/1 -> Altitude PID/1
  max_v_z_mps/1 -> Min/1
  Constant/1 -> Min/2
  Constant1/1 -> Altitude PID/4
  Min/1 -> Gain/1
  Gain/1 -> Altitude PID/5
  P_alt1/1 -> Altitude PID/3
  Altitude PID/1 -> ve_z_cmd/1
  target_z_m/1 -> Sum3/1
  cur_z_m/1 -> Sum3/2

== system malt/PARAM INDEX WAYPOINT CONTROLLER/WP_NAV/heading_controller/heading_controller ==
  heading_cmd_rad : Inport
  <heading_rad> : Inport  Port=2
  D_heading : Constant  Value=Aircraft.Control.D_heading  OutDataTypeStr=single
  Discrete Derivative : simulink/Discrete/Discrete Derivative  gainval=1.0  ICPrevScaledInput=0.0  OutMin=[]  OutMax=[]  OutDataType=fixdt(1, 16)  OutScaling=2^-10  DoSatur=off
  I_heading : Constant  Value=Aircraft.Control.I_heading  OutDataTypeStr=single
  PID Controller2 : slpidlib/PID Controller  Controller=PI  Form=Ideal  TimeDomain=Discrete-time  UseExternalTs=off  SampleTime=framePeriod_s  IntegratorMethod=Forward Euler  FilterMethod=Forward Euler  ControllerParametersSource=external  P=1.85  I=0.01  UseKiTs=off  D=0  N=100  UseFilter=off  TunerSelectOption=Transfer Function Based (PID Tuner App)  InitialConditionSource=internal  InitialConditionForIntegrator=0  InitialConditionForFilter=0  DifferentiatorICPrevScaledInput=0  ExternalReset=none  TrackingMode=off  Kt=1  LimitOutput=on  SatLimitsSource=internal  UpperSaturationLimit=inf  LowerSaturationLimit=-inf  LinearizeAsGain=on  AntiWindupMode=clamping  Kb=2  POutMin=[]  POutMax=[]  IOutMin=[]  IOutMax=[]  DOutMin=[]  DOutMax=[]  NOutMin=[]  NOutMax=[]  SumOutMin=[]  SumOutMax=[]  SaturationOutMin=[]  SaturationOutMax=[]  PParamMin=[]  PParamMax=[]  IParamMin=[]  IParamMax=[]  DParamMin=[]  DParamMax=[]  NParamMin=[]  NParamMax=[]  KbParamMin=[]  KbParamMax=[]  KtParamMin=[]  KtParamMax=[]  KbOutMin=[]  KbOutMax=[]  KtOutMin=[]  KtOutMax=[]  IntegratorOutMin=[]  IntegratorOutMax=[]  FilterOutMin=[]  FilterOutMax=[]  SumI1OutMin=[]  SumI1OutMax=[]  SumI2OutMin=[]  SumI2OutMax=[]  SumI3OutMin=[]  SumI3OutMax=[]  SumI4OutMin=[]  SumI4OutMax=[]  SumDOutMin=[]  SumDOutMax=[]  DifferentiatorOutMin=[]  DifferentiatorOutMax=[]  FilterDiffOutCoefMin=[]  FilterDiffOutCoefMax=[]  ReciprocalOutMin=[]  ReciprocalOutMax=[]  SumDenOutMin=[]  SumDenOutMax=[]  SumNumOutMin=[]  SumNumOutMax=[]  DivideOutMin=[]  DivideOutMax=[]  UdiffTsProdOutMin=[]  UdiffTsProdOutMax=[]  NTsProdOutMin=[]  NTsProdOutMax=[]  UintegralTsProdOutMin=[]  UintegralTsProdOutMax=[]  UngainTsProdOutMin=[]  UngainTsProdOutMax=[]  IntegratorContinuousStateAttributes=''  IntegratorStateMustResolveToSignalObject=off  IntegratorRTWStateStorageClass=Auto  FilterContinuousStateAttributes=''  FilterStateMustResolveToSignalObject=off  FilterRTWStateStorageClass=Auto  ParallelPVariant=Passthrough  IdealPVariant=ExternalParameters  IVariant=ExternalParameters  DVariant=Disabled  IntegratorVariant=Discrete  SatVariant=Enabled  AWVariant=DiscClampingIdeal  PCopyVariant=ExternalParamsIdeal  TRVariant=Disabled  FdbkBlocksVariant=Forward  IdealPFdbkVariant=Disabled  SatFdbkVariant=Disabled  DerivativeFilterVariant=Disabled  NVariant=Disabled  NCopyVariant=Disabled_SignalSpec  FilterICVariant=Disabled  IntegratorICVariant=InternalICs  ExternalResetVariant=Disabled  TRSumVariant=Passthrough  SumFdbkVariant=Disabled  SumVariant=Sum_PI  TsampFilterVariant=InternalTs  TsampNgainVariant=Passthrough  TsampIntegralVariant=Passthrough  ExternalSaturationOutDataTypeStr=Inherit: Same as second input  aMode=0
  P_heading : Constant  Value=Aircraft.Control.P_heading  OutDataTypeStr=single
  Product : Product
  Saturation : Saturate  UpperLimit=Aircraft.Control.yaw_rate_max  LowerLimit=-Aircraft.Control.yaw_rate_max
  Sum : Sum  Inputs=|+-
  heading_error : Subsystem
  yaw_rate_cmd : Outport
  wires:
  P_heading/1 -> PID Controller2/2
  heading_cmd_rad/1 -> heading_error/1(heading_cmd_rad)
  I_heading/1 -> PID Controller2/3
  <heading_rad>/1 -> Discrete Derivative/1, heading_error/2(heading_rad)
  Saturation/1 -> yaw_rate_cmd/1
  heading_error/1(heading_error_rad) -> PID Controller2/1
  Discrete Derivative/1 -> Product/1
  D_heading/1 -> Product/2
  PID Controller2/1 -> Sum/1
  Sum/1 -> Saturation/1
  Product/1 -> Sum/2

== system malt/POS_HOLD CONTROLLER/Horizontal speed controller/Subsystem/roll_D_DLPF ==
  raw_val : Inport
  freq_cut : Inport  Port=2
  Constant : Constant  Value=50  OutDataTypeStr=single
  MATLAB Function : MATLAB Function  TreatAsAtomicUnit=on
  Unit Delay : UnitDelay  SampleTime=-1  HasFrameUpgradeWarning=on
  filtered_val : Outport
  wires:
  freq_cut/1 -> MATLAB Function/3(freq_cut)
  MATLAB Function/1(filtered_val) -> Unit Delay/1, filtered_val/1
  Unit Delay/1 -> MATLAB Function/1(prev_val)
  raw_val/1 -> MATLAB Function/2(raw_val)
  Constant/1 -> MATLAB Function/4(samp_freq)

== system malt/POS_HOLD CONTROLLER/Horizontal speed controller/Subsystem/roll_D_DLPF1 ==
  raw_val : Inport
  freq_cut : Inport  Port=2
  Constant : Constant  Value=50  OutDataTypeStr=single
  MATLAB Function : MATLAB Function  TreatAsAtomicUnit=on
  Unit Delay : UnitDelay  SampleTime=-1  HasFrameUpgradeWarning=on
  filtered_val : Outport
  wires:
  Constant/1 -> MATLAB Function/4(samp_freq)
  raw_val/1 -> MATLAB Function/2(raw_val)
  Unit Delay/1 -> MATLAB Function/1(prev_val)
  MATLAB Function/1(filtered_val) -> filtered_val/1, Unit Delay/1
  freq_cut/1 -> MATLAB Function/3(freq_cut)

== system malt/POS_HOLD CONTROLLER/Horizontal speed controller/Subsystem1/roll_D_DLPF ==
  raw_val : Inport
  freq_cut : Inport  Port=2
  Constant : Constant  Value=50  OutDataTypeStr=single
  MATLAB Function : MATLAB Function  TreatAsAtomicUnit=on
  Unit Delay : UnitDelay  SampleTime=-1  HasFrameUpgradeWarning=on
  filtered_val : Outport
  wires:
  freq_cut/1 -> MATLAB Function/3(freq_cut)
  MATLAB Function/1(filtered_val) -> Unit Delay/1, filtered_val/1
  Unit Delay/1 -> MATLAB Function/1(prev_val)
  raw_val/1 -> MATLAB Function/2(raw_val)
  Constant/1 -> MATLAB Function/4(samp_freq)

== system malt/POS_HOLD CONTROLLER/Horizontal speed controller/Subsystem1/roll_D_DLPF1 ==
  raw_val : Inport
  freq_cut : Inport  Port=2
  Constant : Constant  Value=50  OutDataTypeStr=single
  MATLAB Function : MATLAB Function  TreatAsAtomicUnit=on
  Unit Delay : UnitDelay  SampleTime=-1  HasFrameUpgradeWarning=on
  filtered_val : Outport
  wires:
  Constant/1 -> MATLAB Function/4(samp_freq)
  raw_val/1 -> MATLAB Function/2(raw_val)
  Unit Delay/1 -> MATLAB Function/1(prev_val)
  MATLAB Function/1(filtered_val) -> filtered_val/1, Unit Delay/1
  freq_cut/1 -> MATLAB Function/3(freq_cut)

== system malt/POS_HOLD CONTROLLER/Horizontal speed controller/zero_vel_handling/Horizontal position controller ==
  cur_target_pos_m : Inport
  cur_pos_m : Inport  Port=2
  cur_heading_rad : Inport  Port=3
  P : Inport  Port=4
  Horizontal_position_controller : Subsystem
  "horizontal_error_calculation " : Subsystem
  vb_x_cmd_mps : Outport
  vb_y_cmd_mps : Outport  Port=2
  wires:
  Horizontal_position_controller/1(vb_x) -> vb_x_cmd_mps/1
  Horizontal_position_controller/2(vb_y) -> vb_y_cmd_mps/1
  "horizontal_error_calculation "/1(dist_to_target_m) -> Horizontal_position_controller/1(dist_to_tar_m)
  "horizontal_error_calculation "/2(bearing_to_tar_rad) -> Horizontal_position_controller/2(bearing_to_tar_rad)
  cur_target_pos_m/1 -> "horizontal_error_calculation "/1(target_pos_m)
  cur_pos_m/1 -> "horizontal_error_calculation "/2(cur_pos_m)
  cur_heading_rad/1 -> Horizontal_position_controller/3(cur_heading_rad)
  P/1 -> Horizontal_position_controller/4(P)

== system malt/POS_HOLD CONTROLLER/Horizontal speed controller/zero_vel_handling/set_tar_pos when vel_cmd == 0 ==
  pos_xy_m : Inport
  Enable : EnablePort
  target_pos_xy_m : Outport
  wires:
  pos_xy_m/1 -> target_pos_xy_m/1
